simulink model "model110930"  (R2020a)
settings: Solver=VariableStepAuto  StartTime=0.0  StopTime=8.0  RelTol=1e-3
libraries: commseqgen3 x3
settings Model: Creator=User  LastModifiedBy=User

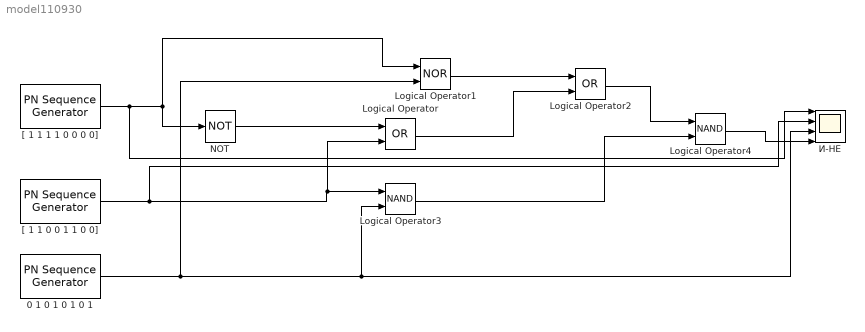
== system model110930 ==
  " 0 1 0 1 0 1 0 1" : commseqgen3/PN Sequence Generator  poly='z^8 + z + 1'  ini_sta=[0 1 0 1 0 1 0 1]  outBitMaskSource=Dialog parameter  shift=0  outVarSiz=off  maxOutSizeMode=Dialog parameter  maxOutSize=[10 1]  Ts=1  sampPerFrame=1  reset=off  bitPackedOutputs=off  outDataType=double  numPackedBits=8  bitPackDataSigned=off  bitPackedOutDType=double
  Logical Operator : Logic  Operator=OR  AllPortsSameDT=off  OutDataTypeStr=boolean
  Logical Operator1 : Logic  Operator=NOR  AllPortsSameDT=off  OutDataTypeStr=boolean
  Logical Operator2 : Logic  Operator=OR  AllPortsSameDT=off  OutDataTypeStr=boolean
  Logical Operator3 : Logic  Operator=NAND  AllPortsSameDT=off  OutDataTypeStr=boolean
  Logical Operator4 : Logic  Operator=NAND  AllPortsSameDT=off  OutDataTypeStr=boolean
  NOT : Logic  Operator=NOT  IconShape=distinctive  AllPortsSameDT=off  OutDataTypeStr=boolean
  "[ 1 1 0 0 1 1 0 0]" : commseqgen3/PN Sequence Generator  poly='z^8 + z + 1'  ini_sta=[0 0 1 1 0 0 1 1]  outBitMaskSource=Dialog parameter  shift=0  outVarSiz=off  maxOutSizeMode=Dialog parameter  maxOutSize=[10 1]  Ts=1  sampPerFrame=1  reset=off  bitPackedOutputs=off  outDataType=double  numPackedBits=8  bitPackDataSigned=off  bitPackedOutDType=double
  "[ 1 1 1 1 0 0 0 0]" : commseqgen3/PN Sequence Generator  poly='z^8 + z + 1'  ini_sta=[ 1 1 1 1 0 0 0 0]  outBitMaskSource=Dialog parameter  shift=0  outVarSiz=off  maxOutSizeMode=Dialog parameter  maxOutSize=[10 1]  Ts=1  sampPerFrame=1  reset=off  bitPackedOutputs=off  outDataType=double  numPackedBits=8  bitPackDataSigned=off  bitPackedOutDType=double
  И-НЕ : Scope  NumInputPorts=4
  wires:
  Logical Operator1/1 -> Logical Operator2/1
  "[ 1 1 1 1 0 0 0 0]"/1 -> И-НЕ/1, NOT/1, Logical Operator1/1
  NOT/1 -> Logical Operator/1
  "[ 1 1 0 0 1 1 0 0]"/1 -> И-НЕ/2, Logical Operator3/1, Logical Operator/2
  " 0 1 0 1 0 1 0 1"/1 -> И-НЕ/3, Logical Operator3/2, Logical Operator1/2
  Logical Operator/1 -> Logical Operator2/2
  Logical Operator2/1 -> Logical Operator4/1
  Logical Operator3/1 -> Logical Operator4/2
  Logical Operator4/1 -> И-НЕ/4
